simulink model "New_control_design"  (R2021a)
settings: Solver=VariableStepAuto  StartTime=0.0  StopTime=10.0  RelTol=1e-3
libraries: simulink x1
settings Model: Creator=20193167  LastModifiedBy=20192670
settings SolverCC: AlgebraicLoopSolver=TrustRegion
settings DebuggingCC: SFMachineParentedDataDiag=warning
settings SFSimCC: CustomCodeUndefinedFunction=UseInterfaceOnly

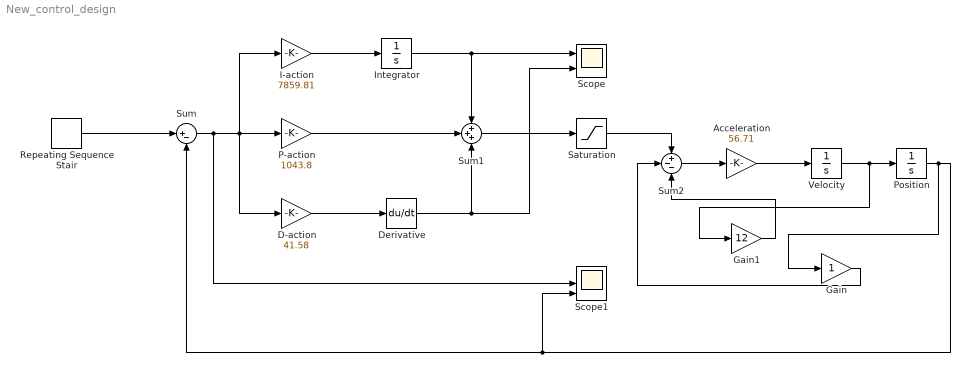
== system New_control_design ==
  Acceleration : Gain  Gain=56.71
  "D-action " : Gain  Gain=41.58
  Derivative : Derivative
  Gain : Gain
  Gain1 : Gain  Gain=12
  "I-action " : Gain  Gain=7859.81
  Integrator : Integrator
  P-action : Gain  Gain=1043.8
  Position : Integrator
  Repeating Sequence Stair : simulink/Sources/Repeating Sequence Stair  OutValues=[1 1 1 1].'  tsamp=-1  OutMin=[]  OutMax=[]  OutDataTypeStr=double  OutputDataTypeScalingMode=double  OutDataType=fixdt(0,8)  ConRadixGroup=Best Precision: Vector-wise  OutScaling=2^-12
  Saturation : Saturate
  Scope : Scope  NumInputPorts=2
  Scope1 : Scope  NumInputPorts=3
  Sum : Sum  Inputs=|+-
  Sum1 : Sum  Inputs=+++
  Sum2 : Sum  Inputs=+--
  Velocity : Integrator
  wires:
  Repeating Sequence Stair/1 -> Sum/1
  Sum/1 -> Scope1/2, "D-action "/1, "I-action "/1, P-action/1
  "I-action "/1 -> Integrator/1
  P-action/1 -> Sum1/2
  "D-action "/1 -> Derivative/1
  Integrator/1 -> Scope/1, Sum1/1
  Derivative/1 -> Scope/2, Sum1/3
  Sum1/1 -> Saturation/1
  Saturation/1 -> Sum2/1
  Sum2/1 -> Acceleration/1
  Acceleration/1 -> Velocity/1
  Velocity/1 -> Gain1/1, Position/1
  Position/1 -> Gain/1, Scope1/3, Sum/2
  Gain/1 -> Sum2/2
  Gain1/1 -> Sum2/3
